simulink model "Android_thingspeak"  (R2018b)
settings: Solver=FixedStepAuto  StartTime=0.0  StopTime=inf  RelTol=1e-3
libraries: androiduilib x11, androidcommunicationlib x4
settings Model: Creator=aelnabty  LastModifiedBy=aelnabty
settings OptimizationCC: EnhancedBackFolding=on  PassReuseOutputArgsAs=Individual arguments  MaxStackSize=64  OptimizeBlockOrder=speed  DifferentSizesBufferReuse=on  OptimizationCustomize=off
settings DebuggingCC: ParameterTunabilityLossMsg=error
settings HardwareCC: ProdBitPerPointer=32  ProdBitPerSizeT=32  ProdBitPerPtrDiffT=32  ProdLargestAtomicInteger=Long  ProdLargestAtomicFloat=Double  ProdWordSize=32  ProdHWDeviceType=ARM Compatible->ARM Cortex
settings SFSimCC: MATLABDynamicMemAlloc=off
settings RTWCC: SystemTargetFile=ert.tlc  HardwareBoard=Android Device  TLCOptions="-aInlineSetEventsForThisBaseRateFcn=TLC_FALSE -aSuppressMultiTaskScheduler=TLC_FALSE  -aRateBasedStepFcn=0"  TemplateMakefile=ert_default_tmf  GenerateReport=on  RTWVerbose=off  Toolchain=Android SDK/NDK Tools  BuildConfiguration=Faster Runs  IncludeHyperlinkInReport=on  LaunchReport=on  GenerateTraceInfo=on  GenerateTraceReport=on  GenerateTraceReportSl=on  GenerateTraceReportSf=on  GenerateTraceReportEml=on
settings CodeAppCC: ForceParamTrailComments=on  IgnoreCustomStorageClasses=off  OperatorAnnotations=on  SimulinkDataObjDesc=on  SFDataObjDesc=on  InsertBlockDesc=on

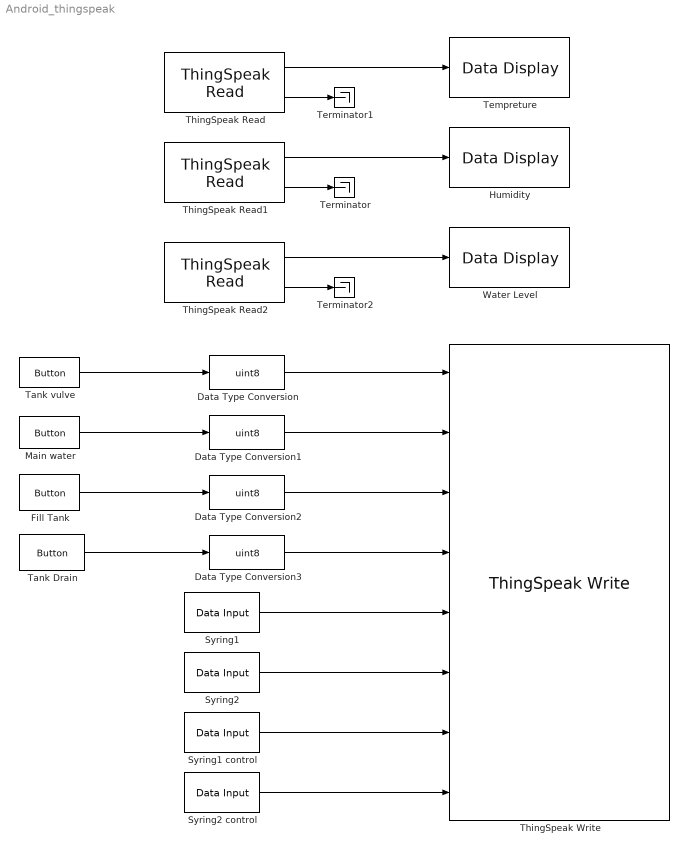
== system Android_thingspeak ==
  Data Type Conversion{,1..3} (4 alike) : DataTypeConversion  OutDataTypeStr=uint8
  Fill Tank : androiduilib/Button  ButtonState=Pressed  ButtonId=Android_thingspeak/Fill_Tank  State=on  SampleTime=0.1  BlockPlatform=Android
      settings: SourceProductName=Simulink Support Package for Android Devices  SourceProductBaseCode=ANDROID
  Humidity : androiduilib/Data Display  DataDisplayId=Android_thingspeak/Humidity  Format=Integer  Precision=6  SimulateUsing=Code generation  blockPlatform=Android
      settings: SourceProductName=Simulink Support Package for Android Devices  SourceProductBaseCode=ANDROID
  Main water : androiduilib/Button  ButtonState=Pressed  ButtonId=Android_thingspeak/Main_water  State=on  SampleTime=0.1  BlockPlatform=Android
      settings: SourceProductName=Simulink Support Package for Android Devices  SourceProductBaseCode=ANDROID
  Syring1 : androiduilib/Data Input  isCharVector=off  Value=1  CharVector=1  OutputDataType=int8  maxCharVectorSize=4  DataInputId=Android_thingspeak/Syring1  SampleTime=0.1
      settings: SourceProductName=Simulink Support Package for Android Devices  SourceProductBaseCode=ANDROID
  Syring1 control : androiduilib/Data Input  isCharVector=off  Value=1  CharVector=1  OutputDataType=int8  maxCharVectorSize=4  DataInputId=Android_thingspeak/Syring1_control  SampleTime=0.1
      settings: SourceProductName=Simulink Support Package for Android Devices  SourceProductBaseCode=ANDROID
  Syring2 : androiduilib/Data Input  isCharVector=off  Value=1  CharVector=1  OutputDataType=int8  maxCharVectorSize=4  DataInputId=Android_thingspeak/Syring2  SampleTime=0.1
      settings: SourceProductName=Simulink Support Package for Android Devices  SourceProductBaseCode=ANDROID
  Syring2 control : androiduilib/Data Input  isCharVector=off  Value=1  CharVector=1  OutputDataType=int8  maxCharVectorSize=4  DataInputId=Android_thingspeak/Syring2_control  SampleTime=0.1
      settings: SourceProductName=Simulink Support Package for Android Devices  SourceProductBaseCode=ANDROID
  Tank Drain : androiduilib/Button  ButtonState=Pressed  ButtonId=Android_thingspeak/Tank_Drain  State=on  SampleTime=0.1  BlockPlatform=Android
      settings: SourceProductName=Simulink Support Package for Android Devices  SourceProductBaseCode=ANDROID
  Tank vulve : androiduilib/Button  ButtonState=Pressed  ButtonId=Android_thingspeak/Tank_vulve  State=on  SampleTime=0.1  BlockPlatform=Android
      settings: SourceProductName=Simulink Support Package for Android Devices  SourceProductBaseCode=ANDROID
  Tempreture : androiduilib/Data Display  DataDisplayId=Android_thingspeak/Tempreture  Format=Integer  Precision=6  SimulateUsing=Code generation  blockPlatform=Android
      settings: SourceProductName=Simulink Support Package for Android Devices  SourceProductBaseCode=ANDROID
  Terminator : Terminator
  Terminator1 : Terminator
  Terminator2 : Terminator
  ThingSpeak Read : androidcommunicationlib/ThingSpeak Read  ChannelID=873337  ChannelAccess=Private  ReadAPIKey=FIG9SNR46R1PTQFB  FieldNumber=1  SampleTime=3  SimulateUsing=Code generation
      settings: SourceProductName=Simulink Support Package for Android Devices  SourceProductBaseCode=ANDROID
  ThingSpeak Read1 : androidcommunicationlib/ThingSpeak Read  ChannelID=873337  ChannelAccess=Private  ReadAPIKey=FIG9SNR46R1PTQFB  FieldNumber=2  SampleTime=3  SimulateUsing=Code generation
      settings: SourceProductName=Simulink Support Package for Android Devices  SourceProductBaseCode=ANDROID
  ThingSpeak Read2 : androidcommunicationlib/ThingSpeak Read  ChannelID=873337  ChannelAccess=Private  ReadAPIKey=FIG9SNR46R1PTQFB  FieldNumber=3  SampleTime=3  SimulateUsing=Code generation
      settings: SourceProductName=Simulink Support Package for Android Devices  SourceProductBaseCode=ANDROID
  ThingSpeak Write : androidcommunicationlib/ThingSpeak Write  ChannelID=903379  WriteAPIKey=D0FYYAJ25YPKUU0I  NumberOfFields=8  UpdateInterval=3  LocationEnabled=off  LocationSource=Block dialog  BlockPlatform=Android
      settings: SourceProductName=Simulink Support Package for Android Devices  SourceProductBaseCode=ANDROID
  Water Level : androiduilib/Data Display  DataDisplayId=Android_thingspeak/Water_Level  Format=Integer  Precision=6  SimulateUsing=Code generation  blockPlatform=Android
      settings: SourceProductName=Simulink Support Package for Android Devices  SourceProductBaseCode=ANDROID
  wires:
  Data Type Conversion1/1 -> ThingSpeak Write/2
  Tank vulve/1 -> Data Type Conversion/1
  Tank Drain/1 -> Data Type Conversion3/1
  Data Type Conversion/1 -> ThingSpeak Write/1
  Data Type Conversion3/1 -> ThingSpeak Write/4
  Main water/1 -> Data Type Conversion1/1
  Data Type Conversion2/1 -> ThingSpeak Write/3
  ThingSpeak Read/1 -> Tempreture/1
  ThingSpeak Read2/1 -> Water Level/1
  Syring1/1 -> ThingSpeak Write/5
  ThingSpeak Read1/1 -> Humidity/1
  Syring2 control/1 -> ThingSpeak Write/8
  Syring1 control/1 -> ThingSpeak Write/7
  ThingSpeak Read1/2 -> Terminator/1
  Syring2/1 -> ThingSpeak Write/6
  ThingSpeak Read/2 -> Terminator1/1
  Fill Tank/1 -> Data Type Conversion2/1
  ThingSpeak Read2/2 -> Terminator2/1
